simulink model "q1"  (R2019a)
settings: Solver=VariableStepAuto  StartTime=0.0  StopTime=100  RelTol=1e-3
values from neighbouring files (symbols this model uses):
  Ka = 4.3    [q1.m]
  m = 1230    [q1.m]
  Vw = 5    [q1.m]
libraries: cstblocks x1
settings Model: Creator=Nir Lalum  LastModifiedBy=Nir Lalum

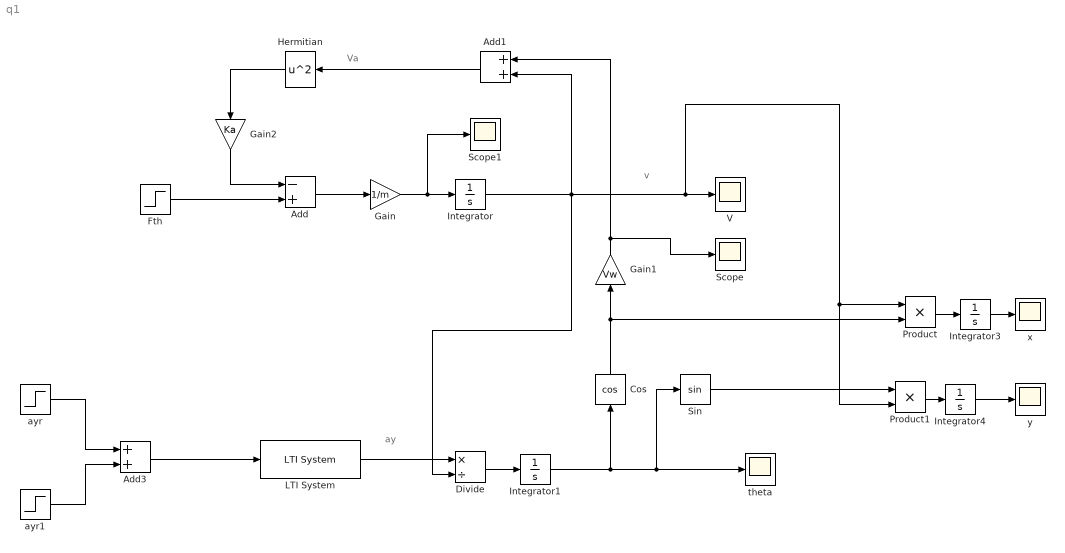
== system q1 ==
  note: v
  note: Va
  note: ay
  Add : Sum  Inputs=-+
  Add1 : Sum
  Add3 : Sum
  Cos : Trigonometry  Operator=cos
  Divide : Product  Inputs=*/
  Fth : Step  Time=0  After=0  SampleTime=0
  Gain : Gain  Gain=1/m
  Gain1 : Gain  Gain=Vw
  Gain2 : Gain  Gain=Ka
  Hermitian : Math  Operator=square  SaturateOnIntegerOverflow=on
  Integrator : Integrator  InitialCondition=40/3.6  LimitOutput=on  UpperSaturationLimit=90/3.6  LowerSaturationLimit=40/3.6
  Integrator1 : Integrator
  Integrator3 : Integrator
  Integrator4 : Integrator
  LTI System : cstblocks/LTI System  sys=G_ayr_ay  IC=[]
  Product : Product
  Product1 : Product
  Scope : Scope
  Scope1 : Scope
  Sin : Trigonometry
  V : Scope
  ayr : Step  Time=0  After=3  SampleTime=0
  ayr1 : Step  Time=70  After=0  SampleTime=0
  theta : Scope
  x : Scope
  y : Scope
  wires:
  Divide/1 -> Integrator1/1
  Cos/1 -> Product/2, Gain1/1
  Fth/1 -> Add/2
  Add/1 -> Gain/1
  Gain1/1 -> Scope/1, Add1/1
  Hermitian/1 -> Gain2/1
  Add1/1 -> Hermitian/1
  LTI System/1 -> Divide/1
  Integrator1/1 -> Cos/1, theta/1, Sin/1
  Gain2/1 -> Add/1
  Gain/1 -> Scope1/1, Integrator/1
  Sin/1 -> Product1/1
  Product/1 -> Integrator3/1
  Product1/1 -> Integrator4/1
  ayr/1 -> Add3/1
  ayr1/1 -> Add3/2
  Integrator/1 -> Product1/2, Product/1, V/1, Divide/2, Add1/2
  Integrator3/1 -> x/1
  Integrator4/1 -> y/1
  Add3/1 -> LTI System/1
